simulink model "car"  (Simulink 7.1)
settings: Solver=ode45  StartTime=0.0  StopTime=10.0  RelTol=1e-3
libraries: fuzblock x1
settings Model: Creator=Renato  LastModifiedBy=Renato
settings DebuggingCC: SaveWithParameterizedLinksMsg=none  SignalResolutionControl=TryResolveAllWithWarning  MultiTaskDSMMsg=warning  MultiTaskCondExecSysMsg=none
settings RTWCC: IncludeERTFirstTime=on
settings GRTTargetCC: TargetFcnLib=ansi_tfl_tmw.mat

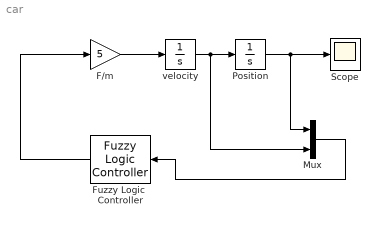
== system car ==
  F/m : Gain  Gain=5  ParameterDataType=sfix(16)  ParameterScaling=2^0  OutDataType=sfix(16)  OutScaling=2^0
  Fuzzy Logic  Controller : fuzblock/Fuzzy Logic  Controller  Orientation=left  SystemSampleTime=-1  fis=car
  Mux : Mux  Inputs=2
  Position : Integrator
  Scope : Scope
      settings: TimeRange=10
  velocity : Integrator  InitialCondition=-3
  wires:
  F/m/1 -> velocity/1
  velocity/1 -> Position/1, Mux/2
  Position/1 -> Scope/1, Mux/1
  Fuzzy Logic  Controller/1 -> F/m/1
  Mux/1 -> Fuzzy Logic  Controller/1
